simulink model "CaseStudyI_9_Bus"  (R2020a)
settings: Solver=FixedStepAuto  StartTime=0.0  StopTime=Tend  FixedStep=T_s_power  MaxStep=5.0E-5  RelTol=1e-3
values from neighbouring files (symbols this model uses):
  B_s46 = b_s46*Cb    (= 9.5071761847e-07)    [Data_CaseStudyI.m]    (also in Data_CaseStudyII.m; Data_InitialSystem.m)
  B_s54 = b_s54*Cb    (= 1.05902722057e-06)    [Data_CaseStudyI.m]    (also in Data_CaseStudyII.m; Data_InitialSystem.m)
  B_s69 = b_s69*Cb    (= 2.15415764185e-06)    [Data_CaseStudyI.m]    (also in Data_CaseStudyII.m; Data_InitialSystem.m)
  B_s75 = b_s75*Cb    (= 1.84126323577e-06)    [Data_CaseStudyI.m]    (also in Data_CaseStudyII.m; Data_InitialSystem.m)
  B_s87 = b_s87*Cb    (= 8.96562817417e-07)    [Data_CaseStudyI.m]    (also in Data_CaseStudyII.m; Data_InitialSystem.m)
  B_s98 = b_s98*Cb    (= 1.25759482443e-06)    [Data_CaseStudyI.m]    (also in Data_CaseStudyII.m; Data_InitialSystem.m)
  C_dc_DVPP_1_2 = 0.008*(n_DVPP_1_2)    (= 0.8)    [Data_CaseStudyI.m]    (also in Data_CaseStudyII.m)
  C_dc_DVPP_1_3 = 0.008*(n_DVPP_1_3)    (= 0.4)    [Data_CaseStudyI.m]    (also in Data_CaseStudyII.m)
  fb = 50    [Data_CaseStudyI.m]    (also in Data_CaseStudyII.m; Data_InitialSystem.m)
  HGov_dyn = HGov_delay*H_tr_droop    [Data_CaseStudyI.m]    (also in Data_CaseStudyII.m; Data_InitialSystem.m)
  HTurb_tot = H_water_way    [Data_CaseStudyI.m]    (also in Data_CaseStudyII.m; Data_InitialSystem.m)
  I_m_DVPP_1_2 = 2/3*Sb_DVPP_1_2/V_m_DVPP_1_2    [Data_CaseStudyI.m]    (also in Data_CaseStudyII.m)
  I_m_DVPP_1_3 = 2/3*Sb_DVPP_1_3/V_m_DVPP_1_3    [Data_CaseStudyI.m]    (also in Data_CaseStudyII.m)
  i_star_max = 1.3    [Data_CaseStudyI.m]    (also in Data_CaseStudyII.m)
  iabc_DVPP_1_2_0 = T0*idq0_DVPP_1_2    [Data_CaseStudyI.m]    (also in Data_CaseStudyII.m)
  iabc_DVPP_1_3_0 = T0*idq0_DVPP_1_3    [Data_CaseStudyI.m]    (also in Data_CaseStudyII.m)
  K2_DVPP_1 = [-0.0221795494247 -1.60799665656 0.160449825826 -2.94803557381 -11.8081988371 -9.75170960256 0.00463021906909 -49.1667298155]    [ControlGains_DVPP1.mat]
  K3_DVPP_1 = [-0.0591512752956 -1.61493903379 -27.2946107927 -16.2119211358 -14.3657419818 2.05688388773 -2.27328406162 0.146700393037 -150.920793597]    [ControlGains_DVPP1.mat]
  k_dc_DVPP_1_2 = eta_DVPP_1_2/(Vdc_n_DVPP_1_2*m_p_DVPP_1_2)    [Data_CaseStudyI.m]    (also in Data_CaseStudyII.m)
  k_dc_DVPP_1_3 = eta_DVPP_1_3/(Vdc_n_DVPP_1_3*m_p_DVPP_1_3)    [Data_CaseStudyI.m]    (also in Data_CaseStudyII.m)
  ki_i_pu = 1.19    [Data_CaseStudyI.m]    (also in Data_CaseStudyII.m)
  ki_pll = 1700    [Data_CaseStudyI.m]    (also in Data_CaseStudyII.m)
  ki_q_pu = 0.005    [Data_CaseStudyI.m]    (also in Data_CaseStudyII.m)
  kp_i_pu = 0.73    [Data_CaseStudyI.m]    (also in Data_CaseStudyII.m)
  kp_pll = 150    [Data_CaseStudyI.m]    (also in Data_CaseStudyII.m)
  kp_q_pu = 0.05    [Data_CaseStudyI.m]    (also in Data_CaseStudyII.m)
  L1_DVPP_1_2_pu = 0.0186/m_DVPP_1_2    (= 0.000372)    [Data_CaseStudyI.m]    (also in Data_CaseStudyII.m)
  L1_DVPP_1_3_pu = 0.0186/m_DVPP_1_3    (= 0.000744)    [Data_CaseStudyI.m]    (also in Data_CaseStudyII.m)
  l1_MVHV1 = 0    [Data_CaseStudyI.m]    (also in Data_CaseStudyII.m; Data_InitialSystem.m)
  l1_MVHV2 = 0    [Data_CaseStudyI.m]    (also in Data_CaseStudyII.m; Data_InitialSystem.m)
  l1_MVHV3 = 0    [Data_CaseStudyI.m]    (also in Data_CaseStudyII.m; Data_InitialSystem.m)
  L2_DVPP_1_2_pu = L1_DVPP_1_2_pu    (= 0.000372)    [Data_CaseStudyI.m]    (also in Data_CaseStudyII.m)
  L2_DVPP_1_3_pu = L1_DVPP_1_3_pu    (= 0.000744)    [Data_CaseStudyI.m]    (also in Data_CaseStudyII.m)
  l2_MVHV1 = l_s14    (= 0.0576)    [Data_CaseStudyI.m]    (also in Data_CaseStudyII.m; Data_InitialSystem.m)
  l2_MVHV2 = l_s72    (= 0.0625)    [Data_CaseStudyI.m]    (also in Data_CaseStudyII.m; Data_InitialSystem.m)
  l2_MVHV3 = l_s39    (= 0.0586)    [Data_CaseStudyI.m]    (also in Data_CaseStudyII.m; Data_InitialSystem.m)
  l_f_DVPP_1_2 = L_f_DVPP_1_2*w_b/Zb_DVPP_1_2    [Data_CaseStudyI.m]    (also in Data_CaseStudyII.m)
  L_f_DVPP_1_2 = (1/(n_DVPP_1_2))*600*10^-6    (= 6e-06)    [Data_CaseStudyI.m]    (also in Data_CaseStudyII.m)
  l_f_DVPP_1_3 = L_f_DVPP_1_3*w_b/Zb_DVPP_1_3    [Data_CaseStudyI.m]    (also in Data_CaseStudyII.m)
  L_f_DVPP_1_3 = (1/(n_DVPP_1_3))*600*10^-6    (= 1.2e-05)    [Data_CaseStudyI.m]    (also in Data_CaseStudyII.m)
  L_s46 = l_s46*Lb    (= 0.154915055408)    [Data_CaseStudyI.m]    (also in Data_CaseStudyII.m; Data_InitialSystem.m)
  L_s54 = l_s54*Lb    (= 0.143128040323)    [Data_CaseStudyI.m]    (also in Data_CaseStudyII.m; Data_InitialSystem.m)
  L_s69 = l_s69*Lb    (= 0.286256080645)    [Data_CaseStudyI.m]    (also in Data_CaseStudyII.m; Data_InitialSystem.m)
  L_s75 = l_s75*Lb    (= 0.271101346964)    [Data_CaseStudyI.m]    (also in Data_CaseStudyII.m; Data_InitialSystem.m)
  L_s87 = l_s87*Lb    (= 0.12123786945)    [Data_CaseStudyI.m]    (also in Data_CaseStudyII.m; Data_InitialSystem.m)
  L_s98 = l_s98*Lb    (= 0.16973301723)    [Data_CaseStudyI.m]    (also in Data_CaseStudyII.m; Data_InitialSystem.m)
  P_L = pL*Sb    (= 300000000)    [Data_CaseStudyI.m]    (also in Data_CaseStudyII.m; Data_InitialSystem.m)
  p_set_bus1 = P_set_bus1/SbSG1    (= 0.731707317073)    [Data_CaseStudyI.m]    (also in Data_CaseStudyII.m; Data_InitialSystem.m)
  p_set_bus2 = P_set_bus2/SbSG2    (= 0.756707317073)    [Data_CaseStudyI.m]    (also in Data_CaseStudyII.m; Data_InitialSystem.m)
  p_set_bus3 = P_set_bus3/SbSG3    (= 0.731707317073)    [Data_CaseStudyI.m]    (also in Data_CaseStudyII.m; Data_InitialSystem.m)
  pset_DVPP_1_1 = P_set_bus1/SbSG1    (= 0.731707317073)    [Data_CaseStudyI.m]    (also in Data_CaseStudyII.m)
  pset_DVPP_1_2 = 0    [Data_CaseStudyI.m]    (also in Data_CaseStudyII.m)
  pset_DVPP_1_3 = 0    [Data_CaseStudyI.m]    (also in Data_CaseStudyII.m)
  Q_L = qL*Sb    (= 82500000)    [Data_CaseStudyI.m]    (also in Data_CaseStudyII.m; Data_InitialSystem.m)
  qset_DVPP_1_2 = 0    [Data_CaseStudyI.m]    (also in Data_CaseStudyII.m)
  qset_DVPP_1_3 = 0    [Data_CaseStudyI.m]    (also in Data_CaseStudyII.m)
  R1_DVPP_1_2_pu = 0.00734/m_DVPP_1_2    (= 0.0001468)    [Data_CaseStudyI.m]    (also in Data_CaseStudyII.m)
  R1_DVPP_1_3_pu = 0.00734/m_DVPP_1_3    (= 0.0002936)    [Data_CaseStudyI.m]    (also in Data_CaseStudyII.m)
  r1_MVHV1 = 1e-6    (= 1e-06)    [Data_CaseStudyI.m]    (also in Data_CaseStudyII.m; Data_InitialSystem.m)
  r1_MVHV2 = 1e-6    (= 1e-06)    [Data_CaseStudyI.m]    (also in Data_CaseStudyII.m; Data_InitialSystem.m)
  r1_MVHV3 = 1e-6    (= 1e-06)    [Data_CaseStudyI.m]    (also in Data_CaseStudyII.m; Data_InitialSystem.m)
  R2_DVPP_1_2_pu = R1_DVPP_1_2_pu    (= 0.0001468)    [Data_CaseStudyI.m]    (also in Data_CaseStudyII.m)
  R2_DVPP_1_3_pu = R1_DVPP_1_3_pu    (= 0.0002936)    [Data_CaseStudyI.m]    (also in Data_CaseStudyII.m)
  r2_MVHV1 = 1e-6    (= 1e-06)    [Data_CaseStudyI.m]    (also in Data_CaseStudyII.m; Data_InitialSystem.m)
  r2_MVHV2 = 1e-6    (= 1e-06)    [Data_CaseStudyI.m]    (also in Data_CaseStudyII.m; Data_InitialSystem.m)
  r2_MVHV3 = 1e-6    (= 1e-06)    [Data_CaseStudyI.m]    (also in Data_CaseStudyII.m; Data_InitialSystem.m)
  R_dc_DVPP_1_2 = (Vdc_n_DVPP_1_2/(0.05*(Sb_DVPP_1_2)/Vdc_n_DVPP_1_2))    [Data_CaseStudyI.m]    (also in Data_CaseStudyII.m)
  R_dc_DVPP_1_3 = (Vdc_n_DVPP_1_3/(0.05*(Sb_DVPP_1_3)/Vdc_n_DVPP_1_3))    [Data_CaseStudyI.m]    (also in Data_CaseStudyII.m)
  r_f_DVPP_1_2 = R_f_DVPP_1_2/Zb_DVPP_1_2    [Data_CaseStudyI.m]    (also in Data_CaseStudyII.m)
  R_f_DVPP_1_2 = 0.02/n_DVPP_1_2    (= 0.0002)    [Data_CaseStudyI.m]    (also in Data_CaseStudyII.m)
  r_f_DVPP_1_3 = R_f_DVPP_1_3/Zb_DVPP_1_3    [Data_CaseStudyI.m]    (also in Data_CaseStudyII.m)
  R_f_DVPP_1_3 = 0.02/n_DVPP_1_3    (= 0.0004)    [Data_CaseStudyI.m]    (also in Data_CaseStudyII.m)
  R_s46 = r_s46*Zb    (= 8.993)    [Data_CaseStudyI.m]    (also in Data_CaseStudyII.m; Data_InitialSystem.m)
  R_s54 = r_s54*Zb    (= 5.29)    [Data_CaseStudyI.m]    (also in Data_CaseStudyII.m; Data_InitialSystem.m)
  R_s69 = r_s69*Zb    (= 20.631)    [Data_CaseStudyI.m]    (also in Data_CaseStudyII.m; Data_InitialSystem.m)
  R_s75 = r_s75*Zb    (= 16.928)    [Data_CaseStudyI.m]    (also in Data_CaseStudyII.m; Data_InitialSystem.m)
  R_s87 = r_s87*Zb    (= 4.4965)    [Data_CaseStudyI.m]    (also in Data_CaseStudyII.m; Data_InitialSystem.m)
  R_s98 = r_s98*Zb    (= 6.2951)    [Data_CaseStudyI.m]    (also in Data_CaseStudyII.m; Data_InitialSystem.m)
  ReferenceSS2_DVPP_1 = ss(M2T_des_DVPP_1,'minimal')    [Data_CaseStudyI.m]    (also in Data_CaseStudyII.m)
  ReferenceSS3_DVPP_1 = ss(M3T_des_DVPP_1,'minimal')    [Data_CaseStudyI.m]    (also in Data_CaseStudyII.m)
  Rg = 0.03    [Data_CaseStudyI.m]    (also in Data_CaseStudyII.m; Data_InitialSystem.m)
  Sb = 100*10^6    (= 100000000)    [Data_CaseStudyI.m]    (also in Data_CaseStudyII.m; Data_InitialSystem.m)
  Sb_DVPP_1_2 = r_b1*100*10^6*cDVPP_1_2    (= 50000000)    [Data_CaseStudyI.m]    (also in Data_CaseStudyII.m)
  Sb_DVPP_1_3 = r_b1*100*10^6*cDVPP_1_3    (= 25000000)    [Data_CaseStudyI.m]    (also in Data_CaseStudyII.m)
  SbSG1 = r_b1*100*10^6    (= 250000000)    [Data_CaseStudyI.m]    (also in Data_CaseStudyII.m; Data_InitialSystem.m)
  SbSG2 = r_b2*100*10^6    (= 96000000)    [Data_CaseStudyI.m]    (also in Data_CaseStudyII.m; Data_InitialSystem.m)
  SbSG3 = r_b3*100*10^6    (= 64000000)    [Data_CaseStudyI.m]    (also in Data_CaseStudyII.m; Data_InitialSystem.m)
  SGov_dyn = tf([1],[Tg 1])    [Data_CaseStudyI.m]    (also in Data_CaseStudyII.m; Data_InitialSystem.m)
  St_MVHV1 = Sb    (= 100000000)    [Data_CaseStudyI.m]    (also in Data_CaseStudyII.m; Data_InitialSystem.m)
  St_MVHV2 = Sb    (= 100000000)    [Data_CaseStudyI.m]    (also in Data_CaseStudyII.m; Data_InitialSystem.m)
  St_MVHV3 = Sb    (= 100000000)    [Data_CaseStudyI.m]    (also in Data_CaseStudyII.m; Data_InitialSystem.m)
  St_MVLV_DVPP_1_2 = St*m_DVPP_1_2    (= 50000000)    [Data_CaseStudyI.m]    (also in Data_CaseStudyII.m)
  St_MVLV_DVPP_1_3 = St*m_DVPP_1_3    (= 25000000)    [Data_CaseStudyI.m]    (also in Data_CaseStudyII.m)
  STurb_reheat = STurb_ch*STurb_rh    [Data_CaseStudyI.m]    (also in Data_CaseStudyII.m; Data_InitialSystem.m)
  T_load_b3 = 2010    [Data_CaseStudyI.m]    (also in Data_CaseStudyII.m = 1010)
  T_load_b6 = 1010    [Data_CaseStudyI.m]    (also in Data_InitialSystem.m)
  T_s_power = 1e-4    (= 0.0001)    [Data_CaseStudyI.m]    (also in Data_CaseStudyII.m; Data_InitialSystem.m)
  tau_dc_DVPP_1_2 = 0.2    [Data_CaseStudyI.m]    (also in Data_CaseStudyII.m)
  tau_dc_DVPP_1_3 = 0.01    [Data_CaseStudyI.m]    (also in Data_CaseStudyII.m)
  V_m_DVPP_1_2 = VbLV_DVPP_1_2*sqrt(2/3)    [Data_CaseStudyI.m]    (also in Data_CaseStudyII.m)
  V_m_DVPP_1_3 = VbLV_DVPP_1_3*sqrt(2/3)    [Data_CaseStudyI.m]    (also in Data_CaseStudyII.m)
  vabc_DVPP_1_2_0_pu = T0*vdq0_DVPP_1_2_0/V_m_DVPP_1_2    [Data_CaseStudyI.m]    (also in Data_CaseStudyII.m)
  vabc_DVPP_1_3_0_pu = T0*vdq0_DVPP_1_3_0/V_m_DVPP_1_3    [Data_CaseStudyI.m]    (also in Data_CaseStudyII.m)
  VbHV = 230*10^3    (= 230000)    [Data_CaseStudyI.m]    (also in Data_CaseStudyII.m; Data_InitialSystem.m)
  VbLV_DVPP_1_2 = 10^3    (= 1000)    [Data_CaseStudyI.m]    (also in Data_CaseStudyII.m)
  VbLV_DVPP_1_3 = 10^3    (= 1000)    [Data_CaseStudyI.m]    (also in Data_CaseStudyII.m)
  VbMV1 = 16.5*10^3    (= 16500)    [Data_CaseStudyI.m]    (also in Data_CaseStudyII.m; Data_InitialSystem.m)
  VbMV2 = 18.0*10^3    (= 18000)    [Data_CaseStudyI.m]    (also in Data_CaseStudyII.m; Data_InitialSystem.m)
  VbMV3 = 13.8*10^3    (= 13800)    [Data_CaseStudyI.m]    (also in Data_CaseStudyII.m; Data_InitialSystem.m)
  vd0_DVPP_1_2_pu = vd0_DVPP_1_2/V_m_DVPP_1_2    [Data_CaseStudyI.m]    (also in Data_CaseStudyII.m)
  vd0_DVPP_1_3_pu = vd0_DVPP_1_3/V_m_DVPP_1_3    [Data_CaseStudyI.m]    (also in Data_CaseStudyII.m)
  Vdc_n_DVPP_1_2 = 3*V_m_DVPP_1_2    [Data_CaseStudyI.m]    (also in Data_CaseStudyII.m)
  Vdc_n_DVPP_1_3 = 3*V_m_DVPP_1_3    [Data_CaseStudyI.m]    (also in Data_CaseStudyII.m)
  w_b = fb*2*pi    (= 314.159265359)    [Data_CaseStudyI.m]    (also in Data_CaseStudyII.m; Data_InitialSystem.m)
  xid0_DVPP_1_2_pu = 0    [Data_CaseStudyI.m]    (also in Data_CaseStudyII.m)
  xid0_DVPP_1_3_pu = 0    [Data_CaseStudyI.m]    (also in Data_CaseStudyII.m)
  xiq0_DVPP_1_2_pu = 0    [Data_CaseStudyI.m]    (also in Data_CaseStudyII.m)
  xiq0_DVPP_1_3_pu = 0    [Data_CaseStudyI.m]    (also in Data_CaseStudyII.m)
  xpll0_pu = w_b/(ki_pll)    (= 0.184799567858)    [Data_CaseStudyI.m]    (also in Data_CaseStudyII.m)
  xq0_DVPP_1_2_pu = xq0_DVPP_1_2/I_m_DVPP_1_2    [Data_CaseStudyI.m]    (also in Data_CaseStudyII.m)
  ... (+1 more)
undefined symbols (not defined in the file or in its folder): A, B, C, Continuous, Dd, Efd0, gcbh, i_dc, Ka, Kf, p2set, SbSM2, sps_rtmsupport, spsST1AModel, Ta, Tb, Tb1, Tc, Tc1, Tf, VA0, VAmax, VAmin, VImax, VImin, VRmax, VRmin
libraries: powerlib x73, powerlib_meascontrol x16, cstblocks x11, sps_avr x2, simulink_extras x1, simulink x1
(part 3 of 3)

== system CaseStudyI_9_Bus/Synchronous Generator 1 Hydro Turbine/Govenor ==
  speed_ref : Inport
  speed : Inport  Port=2
  P_set : Inport  Port=3
  1/droop : Gain  Gain=(-1/Rg)
  Delta speed : Sum  Inputs=-+|
  Govenor Dynamics : cstblocks/LTI System  sys=ss(HGov_dyn)  IC=[1 1.0617]
  Sum : Sum  Inputs=++|
  throttle : Outport  VectorParamsAs1DForOutWhenUnconnected=off
  wires:
  speed/1 -> Delta speed/2
  speed_ref/1 -> Delta speed/1
  Govenor Dynamics/1 -> throttle/1
  Delta speed/1 -> 1/droop/1
  Sum/1 -> Govenor Dynamics/1
  1/droop/1 -> Sum/2  "Pm"
  P_set/1 -> Sum/1

== system CaseStudyI_9_Bus/Synchronous Machine 2 reheat steam turbine/Govenor ==
  speed_ref : Inport
  speed : Inport  Port=2
  P_set : Inport  Port=3
  1/droop : Gain  Gain=(-1/Rg)
  Delta speed : Sum  Inputs=-+|
  Govenor Dynamics : cstblocks/LTI System  sys=ss(SGov_dyn)  IC=[p_set_bus2/2.5]
  Sum : Sum  Inputs=++|
  throttle : Outport  VectorParamsAs1DForOutWhenUnconnected=off
  wires:
  speed/1 -> Delta speed/2
  speed_ref/1 -> Delta speed/1
  Govenor Dynamics/1 -> throttle/1
  Delta speed/1 -> 1/droop/1
  1/droop/1 -> Sum/2  "Pm"
  Sum/1 -> Govenor Dynamics/1
  P_set/1 -> Sum/1

== system CaseStudyI_9_Bus/Synchronous Machine 2 reheat steam turbine/ST1A Excitation System ==
  Vref : Inport
  Vt : Inport  Port=2
  Ifd : Inport  Port=3
  Vstab : Inport  Port=4
  Model : Subsystem  AncestorBlock=spsST1AModel/Continuous  mask(Excitation System){}
  Efd : Outport  VectorParamsAs1DForOutWhenUnconnected=off
  wires:
  Vstab/1 -> Model/4(Vstab)
  Ifd/1 -> Model/3(Ifd)
  Vref/1 -> Model/1(Vref)
  Vt/1 -> Model/2(Vt)
  Model/1(Efd) -> Efd/1

== system CaseStudyI_9_Bus/Synchronous Machine 3 reheat steam turbine/Govenor ==
  speed_ref : Inport
  speed : Inport  Port=2
  P_set : Inport  Port=3
  1/droop : Gain  Gain=(-1/Rg)
  Delta speed : Sum  Inputs=-+|
  Govenor Dynamics : cstblocks/LTI System  sys=ss(SGov_dyn)  IC=[p_set_bus3/2.5]
  Sum : Sum  Inputs=++|
  throttle : Outport  VectorParamsAs1DForOutWhenUnconnected=off
  wires:
  speed/1 -> Delta speed/2
  speed_ref/1 -> Delta speed/1
  Govenor Dynamics/1 -> throttle/1
  Delta speed/1 -> 1/droop/1
  Sum/1 -> Govenor Dynamics/1  "Pm"
  1/droop/1 -> Sum/2
  P_set/1 -> Sum/1

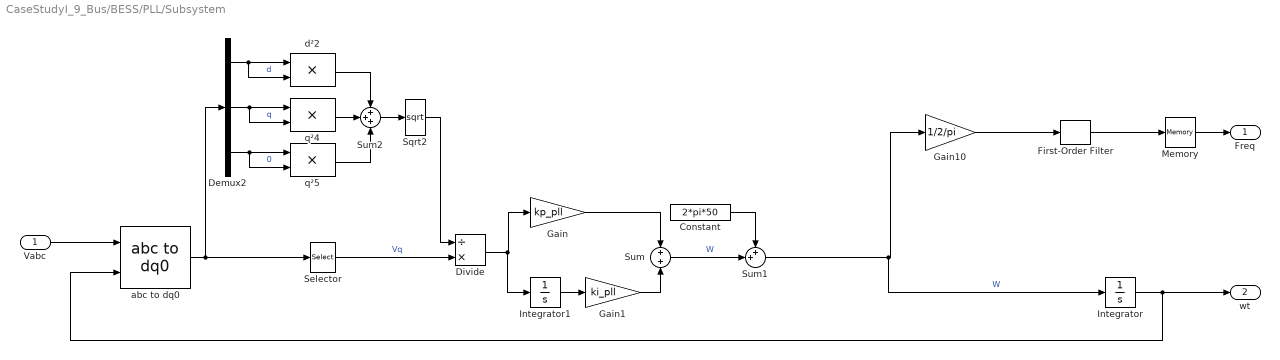
== system CaseStudyI_9_Bus/BESS/PLL/Subsystem ==
  Vabc : Inport  PortDimensions=3
  Constant : Constant  Value=2*pi*50
  Demux2 : Demux  Outputs=3
  Divide : Product  Inputs=/*
  First-Order Filter : powerlib_meascontrol/Filters/First-Order Filter  FilterType=Lowpass  Tc=0.081  Ts=0  Initialize=on  Vac_Init=[0, 0, fb]  Vdc_Init=0  PlotResponse=off  FreqRange="[0,  200,  1]"
  Gain : Gain  Gain=kp_pll
  Gain1 : Gain  Gain=ki_pll
  Gain10 : Gain  Gain=1/2/pi  SaturateOnIntegerOverflow=on  OutDataTypeStr=Inherit: Same as input  ParamDataTypeStr=Inherit: Same as input
  Integrator : Integrator
  Integrator1 : Integrator  InitialCondition=xpll0_pu
  Memory : Memory  InitialCondition=fb
  Selector : Selector  InputPortWidth=3  IndexOptions=Index vector (dialog)  Indices=2  OutputSizes=1
  Sqrt2 : Sqrt  SaturateOnIntegerOverflow=on
  Sum : Sum
  Sum1 : Sum  Inputs=++|
  Sum2 : Sum  Inputs=+++  InputSameDT=on  SaturateOnIntegerOverflow=on  OutDataTypeStr=Inherit: Same as first input
  abc to dq0 : powerlib_meascontrol/Transformations/abc to dq0  Alignment=90 degrees behind phase A axis
      settings: SourceProductBaseCode=MT,PS
  d²2 : Product  InputSameDT=on  RndMeth=Zero  SaturateOnIntegerOverflow=on  OutDataTypeStr=Inherit: Same as first input
  q²4 : Product  InputSameDT=on  RndMeth=Zero  SaturateOnIntegerOverflow=on  OutDataTypeStr=Inherit: Same as first input
  q²5 : Product  InputSameDT=on  RndMeth=Zero  SaturateOnIntegerOverflow=on  OutDataTypeStr=Inherit: Same as first input
  Freq : Outport  VectorParamsAs1DForOutWhenUnconnected=off
  wt : Outport  Port=2  VectorParamsAs1DForOutWhenUnconnected=off
  wires:
  Vabc/1 -> abc to dq0/1
  Integrator/1 -> wt/1, abc to dq0/2
  Memory/1 -> Freq/1
  Gain/1 -> Sum/1
  Gain1/1 -> Sum/2
  Integrator1/1 -> Gain1/1
  Demux2/1 -> d²2/1, d²2/2  "d"
  d²2/1 -> Sum2/1
  Demux2/3 -> q²5/1, q²5/2  "0"
  Demux2/2 -> q²4/1, q²4/2  "q"
  Sqrt2/1 -> Divide/1
  Sum2/1 -> Sqrt2/1
  q²5/1 -> Sum2/3
  abc to dq0/1 -> Demux2/1, Selector/1
  q²4/1 -> Sum2/2
  Selector/1 -> Divide/2  "Vq"
  Divide/1 -> Integrator1/1, Gain/1
  Gain10/1 -> First-Order Filter/1
  First-Order Filter/1 -> Memory/1
  Constant/1 -> Sum1/1
  Sum/1 -> Sum1/2  "W"
  Sum1/1 -> Integrator/1, Gain10/1  "W"

== system CaseStudyI_9_Bus/BESS/Power Controllers/DVPP State Feedback Controller for Active Power Control ==
  P_abc : Inport
  Delta_x_c : Inport  Port=2
  w_pll : Inport  Port=3
  Pset : Inport  Port=4
  Constant : Constant  Value=ReferenceSS2_DVPP_1.A  VectorParams1D=off
  Constant1 : Constant  Value=ReferenceSS2_DVPP_1.B  VectorParams1D=off
  Constant2 : Constant  Value=ReferenceSS2_DVPP_1.C  VectorParams1D=off
  Constant3 : Constant  Value=ReferenceSS2_DVPP_1.D  VectorParams1D=off
  Gain : Gain  Gain=K2_DVPP_1  Multiplication=Matrix(K*u)
  Gain1 : Gain  Gain=1/vd0_DVPP_1_2_pu
  Integrator : Integrator
  Mux : Mux  Inputs=3
  Scope : Scope
  Sum : Sum  Inputs=+-
  Sum1 : Sum  Inputs=++|
  Sum2 : Sum
  Sum3 : Sum  Inputs=-+
  Varying State Space : cstblocks/Linear Parameter Varying/Varying State Space  x0=0  xNames=''  OutputX=on  OutputDX=on
  w* [SI] : Constant
  p_des : Outport
  i_star_d : Outport  Port=2
  wires:
  Mux/1 -> Gain/1
  Varying State Space/1 -> Scope/1, Sum1/2
  Sum3/1 -> Integrator/1
  w* [SI]/1 -> Sum/2
  P_abc/1 -> Sum3/2
  Integrator/1 -> Mux/3
  Varying State Space/2 -> Mux/2
  Delta_x_c/1 -> Mux/1
  w_pll/1 -> Sum/1
  Constant/1 -> Varying State Space/2
  Constant1/1 -> Varying State Space/3
  Constant2/1 -> Varying State Space/4
  Constant3/1 -> Varying State Space/5
  Sum/1 -> Varying State Space/1
  Pset/1 -> Gain1/1, Sum1/1
  Sum1/1 -> Sum3/1, p_des/1
  Sum2/1 -> i_star_d/1
  Gain/1 -> Sum2/1
  Gain1/1 -> Sum2/2

== system CaseStudyI_9_Bus/BESS/Power Controllers/Reactive Power Controller PI-droop control ==
  Q_abc : Inport
  Qset : Inport  Port=2
  Gain : Gain  Gain=kp_q_pu
  Gain1 : Gain  Gain=ki_q_pu
  Integrator1 : Integrator  InitialCondition=xq0_DVPP_1_2_pu
  Sum : Sum  Inputs=-+
  Sum1 : Sum
  i_star_q : Outport
  wires:
  Q_abc/1 -> Sum/2
  Qset/1 -> Sum/1
  Sum/1 -> Integrator1/1, Gain/1
  Gain/1 -> Sum1/1
  Gain1/1 -> Sum1/2
  Integrator1/1 -> Gain1/1
  Sum1/1 -> i_star_q/1

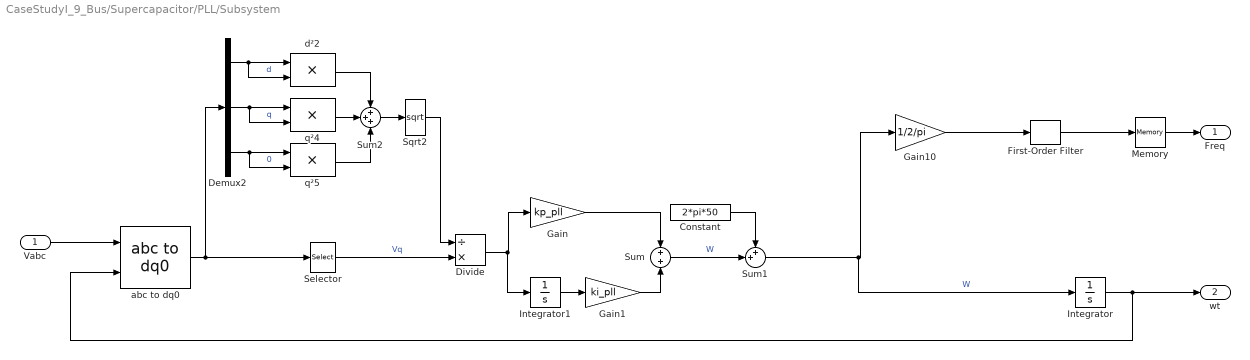
== system CaseStudyI_9_Bus/Supercapacitor/PLL/Subsystem ==
  Vabc : Inport  PortDimensions=3
  Constant : Constant  Value=2*pi*50
  Demux2 : Demux  Outputs=3
  Divide : Product  Inputs=/*
  First-Order Filter : powerlib_meascontrol/Filters/First-Order Filter  FilterType=Lowpass  Tc=0.081  Ts=0  Initialize=on  Vac_Init=[0, 0, fb]  Vdc_Init=0  PlotResponse=off  FreqRange="[0,  200,  1]"
  Gain : Gain  Gain=kp_pll
  Gain1 : Gain  Gain=ki_pll
  Gain10 : Gain  Gain=1/2/pi  SaturateOnIntegerOverflow=on  OutDataTypeStr=Inherit: Same as input  ParamDataTypeStr=Inherit: Same as input
  Integrator : Integrator
  Integrator1 : Integrator  InitialCondition=xpll0_pu
  Memory : Memory  InitialCondition=fb
  Selector : Selector  InputPortWidth=3  IndexOptions=Index vector (dialog)  Indices=2  OutputSizes=1
  Sqrt2 : Sqrt  SaturateOnIntegerOverflow=on
  Sum : Sum
  Sum1 : Sum  Inputs=++|
  Sum2 : Sum  Inputs=+++  InputSameDT=on  SaturateOnIntegerOverflow=on  OutDataTypeStr=Inherit: Same as first input
  abc to dq0 : powerlib_meascontrol/Transformations/abc to dq0  Alignment=90 degrees behind phase A axis
      settings: SourceProductBaseCode=MT,PS
  d²2 : Product  InputSameDT=on  RndMeth=Zero  SaturateOnIntegerOverflow=on  OutDataTypeStr=Inherit: Same as first input
  q²4 : Product  InputSameDT=on  RndMeth=Zero  SaturateOnIntegerOverflow=on  OutDataTypeStr=Inherit: Same as first input
  q²5 : Product  InputSameDT=on  RndMeth=Zero  SaturateOnIntegerOverflow=on  OutDataTypeStr=Inherit: Same as first input
  Freq : Outport  VectorParamsAs1DForOutWhenUnconnected=off
  wt : Outport  Port=2  VectorParamsAs1DForOutWhenUnconnected=off
  wires:
  Vabc/1 -> abc to dq0/1
  Integrator/1 -> wt/1, abc to dq0/2
  Memory/1 -> Freq/1
  Gain/1 -> Sum/1
  Gain1/1 -> Sum/2
  Integrator1/1 -> Gain1/1
  Demux2/1 -> d²2/1, d²2/2  "d"
  d²2/1 -> Sum2/1
  Demux2/3 -> q²5/1, q²5/2  "0"
  Demux2/2 -> q²4/1, q²4/2  "q"
  Sqrt2/1 -> Divide/1
  Sum2/1 -> Sqrt2/1
  q²5/1 -> Sum2/3
  abc to dq0/1 -> Demux2/1, Selector/1
  q²4/1 -> Sum2/2
  Selector/1 -> Divide/2  "Vq"
  Divide/1 -> Integrator1/1, Gain/1
  Gain10/1 -> First-Order Filter/1
  First-Order Filter/1 -> Memory/1
  Constant/1 -> Sum1/1
  Sum/1 -> Sum1/2  "W"
  Sum1/1 -> Integrator/1, Gain10/1  "W"

== system CaseStudyI_9_Bus/Supercapacitor/Power Controllers/DVPP State Feedback Controller for Active Power Control ==
  w_pll : Inport
  P_abc : Inport  Port=2
  Delta_x_c : Inport  Port=3
  P_set : Inport  Port=4
  Constant : Constant  Value=ReferenceSS3_DVPP_1.A  VectorParams1D=off
  Constant1 : Constant  Value=ReferenceSS3_DVPP_1.B  VectorParams1D=off
  Constant2 : Constant  Value=ReferenceSS3_DVPP_1.C  VectorParams1D=off
  Constant3 : Constant  Value=ReferenceSS3_DVPP_1.D  VectorParams1D=off
  Gain : Gain  Gain=K3_DVPP_1  Multiplication=Matrix(K*u)
  Gain1 : Gain
  Gain2 : Gain  Gain=1/vd0_DVPP_1_3_pu
  Integrator : Integrator
  Mux : Mux  Inputs=3
  Scope : Scope
  Sum : Sum  Inputs=+-
  Sum1 : Sum  Inputs=++|
  Sum2 : Sum  Inputs=++|
  Sum3 : Sum  Inputs=-+
  Varying State Space : cstblocks/Linear Parameter Varying/Varying State Space  x0=0  xNames=''  OutputX=on  OutputDX=on
  w* [SI] : Constant
  p_des : Outport
  i_star_d : Outport  Port=2
  wires:
  Mux/1 -> Gain/1
  Varying State Space/1 -> Sum1/2, Scope/1
  Sum3/1 -> Integrator/1
  w_pll/1 -> Gain1/1
  w* [SI]/1 -> Sum/2
  P_abc/1 -> Sum3/2
  Integrator/1 -> Mux/3
  Varying State Space/2 -> Mux/2
  Delta_x_c/1 -> Mux/1
  Gain/1 -> Sum2/1
  Gain1/1 -> Sum/1
  Constant/1 -> Varying State Space/2
  Constant1/1 -> Varying State Space/3
  Constant2/1 -> Varying State Space/4
  Constant3/1 -> Varying State Space/5
  Sum/1 -> Varying State Space/1
  Sum1/1 -> Sum3/1, p_des/1
  P_set/1 -> Gain2/1, Sum1/1
  Gain2/1 -> Sum2/2
  Sum2/1 -> i_star_d/1

== system CaseStudyI_9_Bus/Supercapacitor/Power Controllers/Reactive Power Controller PI-droop control ==
  Q_abc : Inport
  Qset : Inport  Port=2
  Gain : Gain  Gain=kp_q_pu
  Gain1 : Gain  Gain=ki_q_pu
  Integrator1 : Integrator  InitialCondition=xq0_DVPP_1_3_pu
  Sum : Sum  Inputs=-+
  Sum1 : Sum
  i_star_q : Outport
  wires:
  Q_abc/1 -> Sum/2
  Qset/1 -> Sum/1
  Sum/1 -> Integrator1/1, Gain/1
  Gain/1 -> Sum1/1
  Gain1/1 -> Sum1/2
  Integrator1/1 -> Gain1/1
  Sum1/1 -> i_star_q/1

== system CaseStudyI_9_Bus/Synchronous Machine 2 reheat steam turbine/ST1A Excitation System/Model ==
  note: Efd0
  note: Efd0
  note: VA0/Ka
  note: VA0/Ka
  note: Vt.VRmin
  note: VA0/Ka
  note: Efd0
  note: 0
  note: Vt0
  note: Vt.VRmax-Kc.Ifd
  note: Main Regulator
      | Ka/(Ta.s+1)
  note: VImax
  note: Initial values are shown in blue
  note: Vt0
  note: __
      |              /
      |           /
      |         /
      |       /
      | __/
  note: Limits VImin, VImax
  note: VAmax
  note: VAmin
  note: VA0/Ka
  note: KLR*(Ifd-ILR)
  note: VA0=Efd0+KLR*(Ifd-ILR)
  note: VA0
  note: Vt0
  Vref : Inport
  Vt : Inport  Port=2
  Ifd : Inport  Port=3
  Vstab : Inport  Port=4
  Damping Filter Kf.s/(Tf.s+1) : Subsystem  mask(Transfer Function with Initial Outputs){N=[Kf 0], D=[Tf 1], Y0=0, U0=Efd0}
      mask prompts: N "Numerator:"; D "Denominator:"; Y0 "Initial output:"; U0 "Initial input:"
      mask help: Vector expressions for numerator, and denominator. Coefficients are in descending powers of s.
      mask init:
      | [A,B,C,Dd]=tf2ss(N,D);
      | if (isempty(Y0));
      |     [m,n]=size(C);
      |     Y0=zeros(1,m); 
      | end; 
      | if (isempty(U0));
      |     [m,p]=size(B);
      |     U0=zeros(1,p);
      | end;
      | X0=getxo(A,B,C,Dd,U0,Y0,0);
      mask Help: Specify the initial output for the transfer function.  An optimization routine attempts to determine the appropriate initial states so that the specified initial output is achieved.  For more details, see the m-file getxo.m
      mask Display: dpoly(N,D,'s')
  ILR : Constant  Value=ILR
  KLR : Gain  Gain=KLR  SaturateOnIntegerOverflow=on  OutDataTypeStr=Inherit: Same as input  ParamDataTypeStr=Inherit: Same as input
  Low Pass Filter 1/(Tr.s+1) : simulink_extras/Additional Linear/Transfer Fcn (with initial outputs)  N=1  D=[Tr 1]  Y0=Vt0  U0=Vt0
  Subsystem : Subsystem
      mask Display: plot([0.15 0.85],[.5 .5],[.5 .5],[0.05 0.95],0.15+0.7*[0 .25 .75 1],0.05+0.9*[.25 .25 .75 .75]);
  Subtract : Sum  Inputs=+-
  Sum : Sum  Inputs=++-+-  InputSameDT=on  SaturateOnIntegerOverflow=on  OutDataTypeStr=Inherit: Same as first input
  Sum1 : Sum  Inputs=|+-  InputSameDT=on  SaturateOnIntegerOverflow=on  OutDataTypeStr=Inherit: Same as first input
  Sum2 : Sum  Inputs=|+-  InputSameDT=on  SaturateOnIntegerOverflow=on  OutDataTypeStr=Inherit: Same as first input
  Transient Gain Reduction (Tc.s+1).(Tc1.s+1) ----------------------- (Tb.s+1).(Tb1.s+1) : Subsystem  mask(Transfer Function with Initial Outputs){N=[Tc*Tc1 Tc+Tc1 1], D=[Tb*Tb1 Tb+Tb1 1], Y0=VA0/Ka, U0=VA0/Ka}
      mask prompts: N "Numerator:"; D "Denominator:"; Y0 "Initial output:"; U0 "Initial input:"
      mask help: Vector expressions for numerator, and denominator. Coefficients are in descending powers of s.
      mask init:
      | [A,B,C,Dd]=tf2ss(N,D);if (isempty(Y0));[m,n]=size(A);X0=zeros(1,m); end; if (isempty(U0));[m,p]=size(B);U0=zeros(1,p);end;
      |  if isempty(A),  X0=[]; else ,X0=getxo(A,B,C,Dd,U0,Y0,0); end
      mask Help: Specify the initial output for the transfer function.  An optimization routine attempts to determine the appropriate initial states so that the specified initial output is achieved.  For more details, see the m-file getxo.m
      mask Display: dpoly(N,D,'s')
  VA0/Ka : Constant  Value=VA0/Ka
  VImin : Saturate  UpperLimit=VImax  LowerLimit=VImin
  VImin2 : Saturate  UpperLimit=inf  LowerLimit=0
  Vaminmax : Subsystem  mask{Ka=Ka, Ta=Ta, VAminmax=[VAmin VAmax], X0=VA0}
      mask prompts: Ka "Voltage regulator gain Ka:"; Ta "Voltage regulator time constant Ta(s):"; VAminmax "Voltage regulator internal limits [VAmin(pu) VAmax(pu)]:"; X0 "Initial conditions:"
      mask init:
      | VAmin=VAminmax(1);VAmax=VAminmax(2);
      mask Display: dpoly([Ka],[Ta 1],'s')
  Efd : Outport
  wires:
  Ifd/1 -> Sum1/1, Subsystem/3(Ifd)
  Subsystem/1(Efd1) -> Efd/1  "Efd"
  Vt/1 -> Low Pass Filter 1/(Tr.s+1)/1  "Vt"
  Vaminmax/1(y) -> Sum2/1  "VA"
  Sum/1 -> VImin/1
  Sum1/1 -> KLR/1
  ILR/1 -> Sum1/2
  Sum2/1 -> Damping Filter Kf.s/(Tf.s+1)/1(In1), Subsystem/1(Efd)  "Efd"
  Transient Gain Reduction (Tc.s+1).(Tc1.s+1) ----------------------- (Tb.s+1).(Tb1.s+1)/1(Out1) -> Vaminmax/1(u)
  KLR/1 -> VImin2/1
  VA0/Ka/1 -> Sum/2
  Low Pass Filter 1/(Tr.s+1)/1 -> Subtract/2, Subsystem/2(Vt)  "Vt"
  VImin2/1 -> Sum2/2
  Damping Filter Kf.s/(Tf.s+1)/1(Out1) -> Sum/5  "Vf"
  VImin/1 -> Transient Gain Reduction (Tc.s+1).(Tc1.s+1) ----------------------- (Tb.s+1).(Tb1.s+1)/1(In1)  "VI"
  Vstab/1 -> Sum/4
  Vref/1 -> Subtract/1
  Subtract/1 -> Sum/1

== system CaseStudyI_9_Bus/Synchronous Machine 2 reheat steam turbine/ST1A Excitation System/Model/Damping Filter Kf.s//(Tf.s+1) ==
  In1 : Inport
  State Space : StateSpace  A=A  B=B  C=C  D=Dd  InitialCondition=X0
  Out1 : Outport  InitialOutput=0
  wires:
  In1/1 -> State Space/1
  State Space/1 -> Out1/1

== system CaseStudyI_9_Bus/Synchronous Machine 2 reheat steam turbine/ST1A Excitation System/Model/Subsystem ==
  note: Vt.VRmax-Kc.Ifd
  note: Vt.VRmin
  Efd : Inport
  Vt : Inport  Port=2
  Ifd : Inport  Port=3
  Gain2 : Gain  Gain=Kc  SaturateOnIntegerOverflow=on  OutDataTypeStr=Inherit: Same as input  ParamDataTypeStr=Inherit: Same as input
  Gain5 : Gain  Gain=VRmax  SaturateOnIntegerOverflow=on  OutDataTypeStr=Inherit: Same as input  ParamDataTypeStr=Inherit: Same as input
  Gain6 : Gain  Gain=VRmin  SaturateOnIntegerOverflow=on  OutDataTypeStr=Inherit: Same as input  ParamDataTypeStr=Inherit: Same as input
  Saturation Dynamic : simulink/Discontinuities/Saturation Dynamic  OutMin=[]  OutMax=[]  OutDataTypeStr=Inherit: Same as second input  OutDataType=fixdt(1, 16)  OutScaling=2^-10  DoSatur=off
  Sum5 : Sum  Inputs=+-  InputSameDT=on  SaturateOnIntegerOverflow=on  OutDataTypeStr=Inherit: Same as first input
  Efd1 : Outport
  wires:
  Gain2/1 -> Sum5/2
  Ifd/1 -> Gain2/1  "Field current Ifd (pu)"
  Efd/1 -> Saturation Dynamic/2  "Field voltage Efd (pu)"
  Gain6/1 -> Saturation Dynamic/3
  Saturation Dynamic/1 -> Efd1/1
  Gain5/1 -> Sum5/1
  Vt/1 -> Gain6/1, Gain5/1  "Terminal voltage Vt (pu)"
  Sum5/1 -> Saturation Dynamic/1

== system CaseStudyI_9_Bus/Synchronous Machine 2 reheat steam turbine/ST1A Excitation System/Model/Transient Gain Reduction (Tc.s+1).(Tc1.s+1) ----------------------- (Tb.s+1).(Tb1.s+1) ==
  In1 : Inport
  State Space : StateSpace  A=A  B=B  C=C  D=Dd  InitialCondition=X0
  Out1 : Outport  InitialOutput=0
  wires:
  In1/1 -> State Space/1
  State Space/1 -> Out1/1

== system CaseStudyI_9_Bus/Synchronous Machine 2 reheat steam turbine/ST1A Excitation System/Model/Vaminmax ==
  note: VA0/Ka
  note: VA0
  note: VA0
  note: 0
  note: VA0
  u : Inport
  Gain1 : Gain  Gain=1/Ta  SaturateOnIntegerOverflow=on  OutDataTypeStr=Inherit: Same as input  ParamDataTypeStr=Inherit: Same as input
  Gain2 : Gain  Gain=Ka  SaturateOnIntegerOverflow=on  OutDataTypeStr=Inherit: Same as input  ParamDataTypeStr=Inherit: Same as input
  Integrator : Integrator  InitialCondition=VA0  LimitOutput=on  UpperSaturationLimit=VAmax  LowerSaturationLimit=VAmin
  Sum : Sum  Inputs=|+-  InputSameDT=on  SaturateOnIntegerOverflow=on  OutDataTypeStr=Inherit: Same as first input
  y : Outport
  wires:
  u/1 -> Gain2/1
  Sum/1 -> Gain1/1
  Integrator/1 -> y/1, Sum/2
  Gain2/1 -> Sum/1
  Gain1/1 -> Integrator/1
